simulink model "akz_ab1"  (Simulink 4.00)
settings: Solver=ode23  SolverMode=SingleTasking  StartTime=0.0  StopTime=80  RelTol=1e-4  AbsTol=1e-8
libraries: simulink3 x1
CloseFcn:
  | ;slview('closediagram',bdroot);
settings Model: LimitDataPoints=off  BlockReductionOpt=off

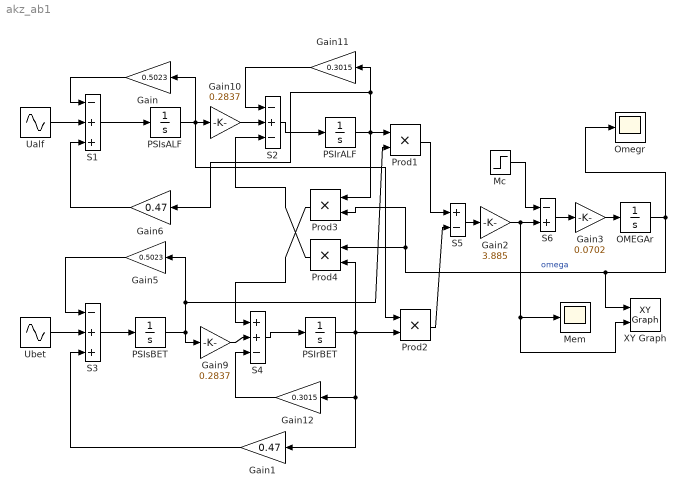
== system akz_ab1 ==
  "  Prod1" : Product  Inputs=2  Multiplication=Element-wise(.*)  SaturateOnIntegerOverflow=on
  Gain : Gain  Orientation=left  Gain=0.5023  Multiplication=Element-wise(K.*u)  SaturateOnIntegerOverflow=on
  Gain1 : Gain  Orientation=left  Gain=0.47  Multiplication=Element-wise(K.*u)  SaturateOnIntegerOverflow=on
  Gain10 : Gain  Gain=0.2837  Multiplication=Element-wise(K.*u)  SaturateOnIntegerOverflow=on
  Gain11 : Gain  Orientation=left  Gain=0.3015  Multiplication=Element-wise(K.*u)  SaturateOnIntegerOverflow=on
  Gain12 : Gain  Orientation=left  Gain=0.3015  Multiplication=Element-wise(K.*u)  SaturateOnIntegerOverflow=on
  Gain2 : Gain  Gain=3.885  Multiplication=Element-wise(K.*u)  SaturateOnIntegerOverflow=on
  Gain3 : Gain  Gain=0.0702  Multiplication=Element-wise(K.*u)  SaturateOnIntegerOverflow=on
  Gain5 : Gain  Orientation=left  Gain=0.5023  Multiplication=Element-wise(K.*u)  SaturateOnIntegerOverflow=on
  Gain6 : Gain  Orientation=left  Gain=0.47  Multiplication=Element-wise(K.*u)  SaturateOnIntegerOverflow=on
  Gain9 : Gain  Gain=0.2837  Multiplication=Element-wise(K.*u)  SaturateOnIntegerOverflow=on
  Mc : Step  Time=0.5  Before=0.0  After=0.33  SampleTime=0
  Mem : Scope
      settings: TickLabels=on  TimeRange=80  YMin=-1  YMax=2  SaveToWorkspace=off  SaveName=ScopeData  DataFormat=Array  MaxDataPoints=5000
  OMEGAr : Integrator  ExternalReset=none  InitialConditionSource=internal  InitialCondition=0  LimitOutput=off  UpperSaturationLimit=inf  LowerSaturationLimit=-inf  ShowSaturationPort=off  ShowStatePort=off  AbsoluteTolerance=auto
  Omegr : Scope
      settings: TickLabels=on  TimeRange=80  YMin=0  YMax=1.4  SaveToWorkspace=off  DataFormat=Array  MaxDataPoints=5000
  PSIrALF : Integrator  ExternalReset=none  InitialConditionSource=internal  InitialCondition=0  LimitOutput=off  UpperSaturationLimit=inf  LowerSaturationLimit=-inf  ShowSaturationPort=off  ShowStatePort=off  AbsoluteTolerance=auto
  PSIrBET : Integrator  ExternalReset=none  InitialConditionSource=internal  InitialCondition=0  LimitOutput=off  UpperSaturationLimit=inf  LowerSaturationLimit=-inf  ShowSaturationPort=off  ShowStatePort=off  AbsoluteTolerance=auto
  PSIsALF : Integrator  ExternalReset=none  InitialConditionSource=internal  InitialCondition=0  LimitOutput=off  UpperSaturationLimit=inf  LowerSaturationLimit=-inf  ShowSaturationPort=off  ShowStatePort=off  AbsoluteTolerance=auto
  PSIsBET : Integrator  ExternalReset=none  InitialConditionSource=internal  InitialCondition=0  LimitOutput=off  UpperSaturationLimit=inf  LowerSaturationLimit=-inf  ShowSaturationPort=off  ShowStatePort=off  AbsoluteTolerance=auto
  Prod2 : Product  Inputs=2  Multiplication=Element-wise(.*)  SaturateOnIntegerOverflow=on
  Prod3 : Product  Orientation=left  Inputs=2  Multiplication=Element-wise(.*)  SaturateOnIntegerOverflow=on
  Prod4 : Product  Orientation=left  Inputs=2  Multiplication=Element-wise(.*)  SaturateOnIntegerOverflow=on
  S1 : Sum  Inputs=-++  SaturateOnIntegerOverflow=on
  S2 : Sum  Inputs=-+-  SaturateOnIntegerOverflow=on
  S3 : Sum  Inputs=-++  SaturateOnIntegerOverflow=on
  S4 : Sum  Inputs=++-  SaturateOnIntegerOverflow=on
  S5 : Sum  Inputs=+-  SaturateOnIntegerOverflow=on
  S6 : Sum  Inputs=-+  SaturateOnIntegerOverflow=on
  Ualf : Sin  Amplitude=1  Frequency=1  Phase=pi/2  SampleTime=0
  Ubet : Sin  Amplitude=1  Frequency=1  Phase=0  SampleTime=0
  XY Graph : simulink3/Sinks/XY Graph  xmin=-0.1  xmax=1.2  ymin=-0.1  ymax=1.8  st=-1
  wires:
  Gain/1 -> S1/1
  S3/1 -> PSIsBET/1
  PSIrBET/1 -> Prod4/2, Prod2/2, Gain1/1, Gain12/1
  PSIrALF/1 -> Prod3/1, "  Prod1"/1, Gain6/1, Gain11/1
  Prod2/1 -> S5/2
  S6/1 -> Gain3/1
  Gain3/1 -> OMEGAr/1
  Mc/1 -> S6/1
  Gain1/1 -> S3/3
  "  Prod1"/1 -> S5/1
  S2/1 -> PSIrALF/1
  S4/1 -> PSIrBET/1
  S5/1 -> Gain2/1
  S1/1 -> PSIsALF/1
  PSIsBET/1 -> Gain9/1, "  Prod1"/2, Gain5/1
  PSIsALF/1 -> Prod2/1, Gain10/1, Gain/1
  Ualf/1 -> S1/2
  Ubet/1 -> S3/2
  Gain10/1 -> S2/2
  Gain9/1 -> S4/2
  Gain6/1 -> S1/3
  Gain5/1 -> S3/1
  Prod4/1 -> S2/3
  Prod3/1 -> S4/1
  Gain2/1 -> S6/2, Mem/1, XY Graph/2
  Gain11/1 -> S2/1
  Gain12/1 -> S4/3
  OMEGAr/1 -> Omegr/1, Prod4/1, Prod3/2, XY Graph/1  "omega"
